simulink subsystem "Drag_Compensator_mk1"  (R2023a)
settings: Solver=VariableStepAuto  StartTime=0.0  StopTime=10.0  RelTol=1e-3
libraries: ros2lib x2

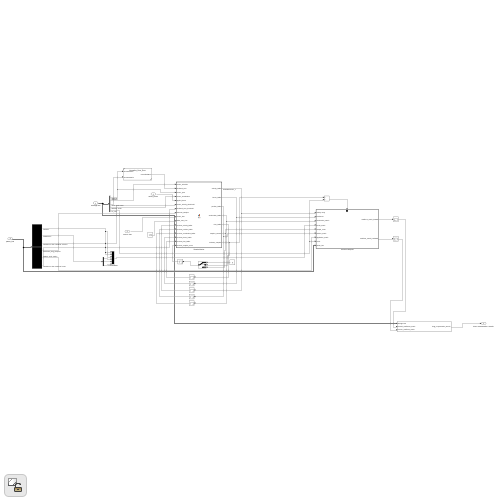
[thumbnail: Simulink's stored preview of the top-level diagram]
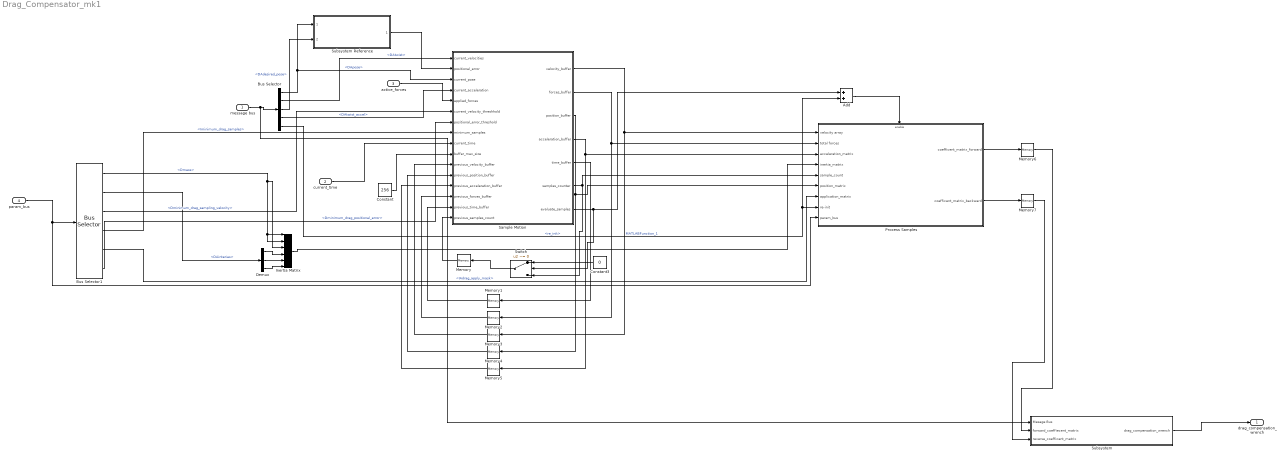
== system Drag_Compensator_mk1 ==
  message bus : Inport
  current_time : Inport  Port=2
  active_forces : Inport  Port=3
  param_bus : Inport  Port=4
  Add : Sum
  Bus Selector : BusSelector  OutputSignals=current_state.DApose,current_state.DAtwist,desired_pose.DAdesired_pose,current_state.DAtwist_accel,re_init
  Bus Selector1 : BusSelector  OutputSignals=Dmass,DAinterias,Dminimum_drag_sampling_velocity,Iminimum_drag_samples,IAdrag_apply_mask,Dminimum_drag_positional_error
  Constant : Constant  Value=256
  Constant3 : Constant  Value=0
  Demux : Demux  Outputs=3
  Inertia Matrix : Mux  Inputs=6
  Memory : Memory
  Memory1 : Memory  InitialCondition=zeros(256,1)
  Memory2 : Memory  InitialCondition=zeros(6,256)
  Memory3 : Memory  InitialCondition=zeros(6,256)
  Memory4 : Memory  InitialCondition=zeros(7,256)
  Memory5 : Memory  InitialCondition=zeros(6,256)
  Memory6 : Memory  InitialCondition=zeros(6,6)
  Memory7 : Memory  InitialCondition=zeros(6,6)
  Process Samples : Subsystem
  Sample Motion : MATLAB Function  TreatAsAtomicUnit=on
  Subsystem : Subsystem
  Subsystem Reference : Subsystem  ReferencedSubsystem=Normalize_Pose_Error
  Switch : Switch  Criteria=u2 ~= 0  SaturateOnIntegerOverflow=off  InputSameDT=off
  drag_compensation_wrench : Outport
  wires:
  Sample Motion/1(velocity_buffer) -> Process Samples/1(velocity array), Memory3/1  "MATLABFunction_1"
  Sample Motion/5(time_buffer) -> Memory1/1
  Sample Motion/6(samples_counter) -> Process Samples/5(sample_count), Switch/3
  Sample Motion/2(forces_buffer) -> Process Samples/2(total forces), Memory2/1
  message bus/1 -> Bus Selector/1, Subsystem/1(Mesage Bus)
  current_time/1 -> Sample Motion/9(current_time)
  Constant/1 -> Sample Motion/10(buffer_max_size)
  Bus Selector/2 -> Sample Motion/1(current_velocities)  "<DAtwist>"
  active_forces/1 -> Sample Motion/5(applied_forces)
  Bus Selector/1 -> Sample Motion/3(current_pose), Subsystem Reference/1  "<DApose>"
  Bus Selector/3 -> Subsystem Reference/2  "<DAdesired_pose>"
  Subsystem Reference/1 -> Sample Motion/2(positional_error)
  Constant3/1 -> Switch/1
  Sample Motion/7(evaluate_samples) -> Add/1, Switch/2
  Switch/1 -> Memory/1
  Memory/1 -> Sample Motion/16(previous_samples_count)
  Memory1/1 -> Sample Motion/15(previous_time_buffer)
  Memory2/1 -> Sample Motion/14(previous_forces_buffer)
  Memory3/1 -> Sample Motion/11(previous_velocity_buffer)
  Sample Motion/3(position_buffer) -> Process Samples/6(position_matrix), Memory4/1
  Memory4/1 -> Sample Motion/12(previous_position_buffer)
  Sample Motion/4(acceleration_buffer) -> Process Samples/3(acceleration_matrix), Memory5/1
  Memory5/1 -> Sample Motion/13(previous_acceleration_buffer)
  Bus Selector/4 -> Sample Motion/4(current_acceleration)  "<DAtwist_accel>"
  param_bus/1 -> Bus Selector1/1, Process Samples/9(param_bus)
  Bus Selector1/2 -> Demux/1  "<DAinterias>"
  Demux/3 -> Inertia Matrix/6
  Demux/2 -> Inertia Matrix/5
  Demux/1 -> Inertia Matrix/4
  Bus Selector1/1 -> Inertia Matrix/3, Inertia Matrix/1, Inertia Matrix/2  "<Dmass>"
  Inertia Matrix/1 -> Process Samples/4(inertia_matrix)
  Process Samples/1(coefficent_matrix_forward) -> Memory6/1
  Bus Selector1/3 -> Sample Motion/6(current_velocity_threshhold)  "<Dminimum_drag_sampling_velocity>"
  Bus Selector1/6 -> Sample Motion/7(positional_error_threshold)  "<Dminimum_drag_positional_error>"
  Bus Selector1/5 -> Process Samples/7(application_matrix)  "<IAdrag_apply_mask>"
  Bus Selector1/4 -> Sample Motion/8(minimum_samples)  "<Iminimum_drag_samples>"
  Bus Selector/5 -> Process Samples/8(re-init), Add/2  "<re_init>"
  Add/1 -> Process Samples/Enable
  Process Samples/2(coefficent_matrix_backward) -> Memory7/1
  Memory6/1 -> Subsystem/2(forward_coeffiecent_matrix)
  Memory7/1 -> Subsystem/3(reverse_coefficent_matrix)
  Subsystem/1(drag_compensation_wrench) -> drag_compensation_wrench/1

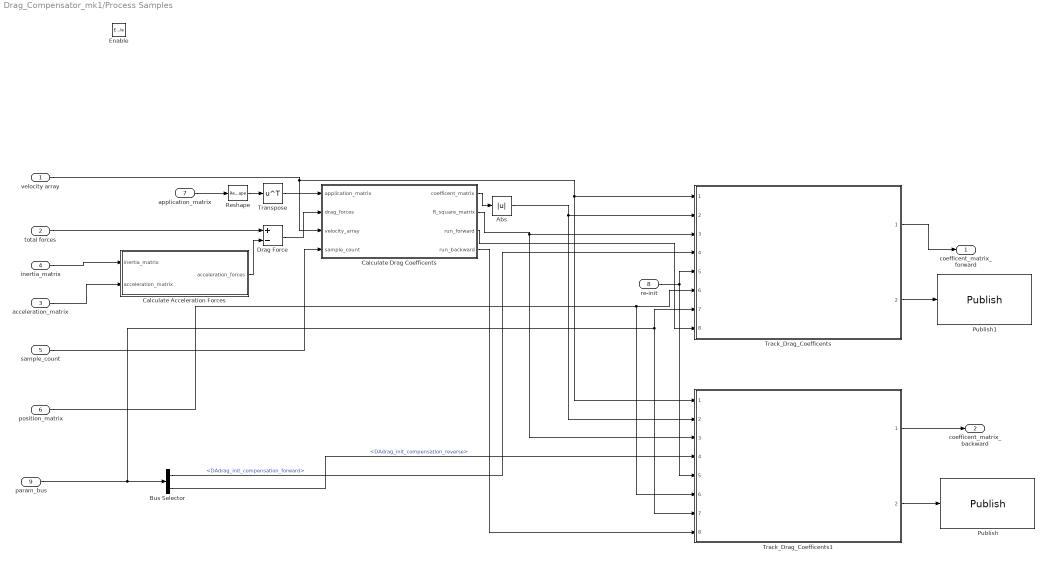
== system Drag_Compensator_mk1/Process Samples ==
  velocity array : Inport
  total forces : Inport  Port=2
  acceleration_matrix : Inport  Port=3
  inertia_matrix : Inport  Port=4
  sample_count : Inport  Port=5
  position_matrix : Inport  Port=6
  application_matrix : Inport  Port=7
  re-init : Inport  Port=8
  param_bus : Inport  Port=9
  Enable : EnablePort
  Abs : Abs  SaturateOnIntegerOverflow=off
  Bus Selector : BusSelector  OutputSignals=DAdrag_init_compensation_forward,DAdrag_init_compensation_reverse
  Calculate Acceleration Forces : MATLAB Function  TreatAsAtomicUnit=on
  Calculate Drag Coefficents : MATLAB Function  TreatAsAtomicUnit=on
  Drag Force : Sum  Inputs=+-
  Publish : ros2lib/Publish  topicSource=Specify your own  topic=/talos/controller/drag_comp/reverse  messageType=geometry_msgs/TwistWithCovariance  QOSHistory=Keep last  QOSDepth=1  QOSReliability=Reliable  QOSDurability=Volatile
  Publish1 : ros2lib/Publish  topicSource=Specify your own  topic=/talos/controller/drag_comp/forward  messageType=geometry_msgs/TwistWithCovariance  QOSHistory=Keep last  QOSDepth=1  QOSReliability=Reliable  QOSDurability=Volatile
  Reshape : Reshape  OutputDimensionality=Customize  OutputDimensions=[6,6]
  Track_Drag_Coefficents : Subsystem  ReferencedSubsystem=Track_Drag_Coefficents
  Track_Drag_Coefficents1 : Subsystem  ReferencedSubsystem=Track_Drag_Coefficents
  Transpose : Math  Operator=transpose
  coefficent_matrix_forward : Outport
  coefficent_matrix_backward : Outport  Port=2
  wires:
  Track_Drag_Coefficents/2 -> Publish1/1
  Track_Drag_Coefficents1/2 -> Publish/1
  Track_Drag_Coefficents1/1 -> coefficent_matrix_backward/1
  Calculate Drag Coefficents/4(run_backward) -> Track_Drag_Coefficents1/8
  Calculate Drag Coefficents/3(run_forward) -> Track_Drag_Coefficents/8
  Bus Selector/2 -> Track_Drag_Coefficents1/4  "<DAdrag_init_compensation_reverse>"
  Bus Selector/1 -> Track_Drag_Coefficents/4  "<DAdrag_init_compensation_forward>"
  param_bus/1 -> Track_Drag_Coefficents/7, Track_Drag_Coefficents1/7, Bus Selector/1
  Track_Drag_Coefficents/1 -> coefficent_matrix_forward/1
  position_matrix/1 -> Track_Drag_Coefficents/6, Track_Drag_Coefficents1/6
  re-init/1 -> Track_Drag_Coefficents/5, Track_Drag_Coefficents1/5
  Calculate Drag Coefficents/2(R_square_matrix) -> Track_Drag_Coefficents/3, Track_Drag_Coefficents1/3
  Abs/1 -> Track_Drag_Coefficents/2, Track_Drag_Coefficents1/2
  Transpose/1 -> Calculate Drag Coefficents/1(application_matrix)
  Reshape/1 -> Transpose/1
  velocity array/1 -> Track_Drag_Coefficents/1, Track_Drag_Coefficents1/1, Calculate Drag Coefficents/3(velocity_array)
  Calculate Drag Coefficents/1(coefficent_matrix) -> Abs/1
  sample_count/1 -> Calculate Drag Coefficents/4(sample_count)
  inertia_matrix/1 -> Calculate Acceleration Forces/1(inertia_matrix)
  total forces/1 -> Drag Force/1
  acceleration_matrix/1 -> Calculate Acceleration Forces/2(acceleration_matrix)
  Drag Force/1 -> Calculate Drag Coefficents/2(drag_forces)
  Calculate Acceleration Forces/1(acceleration_forces) -> Drag Force/2
  application_matrix/1 -> Reshape/1

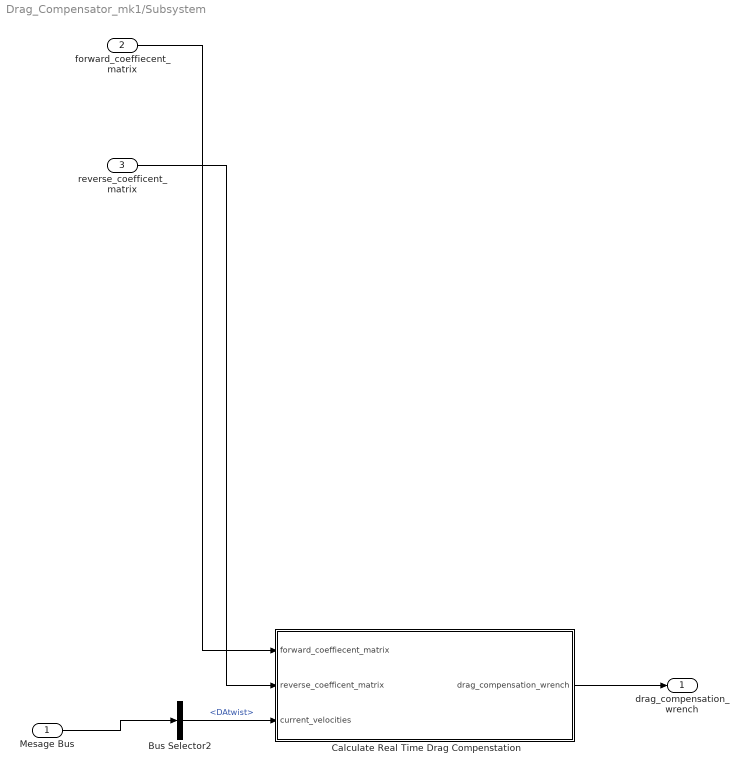
== system Drag_Compensator_mk1/Subsystem ==
  Mesage Bus : Inport
  forward_coeffiecent_matrix : Inport  Port=2
  reverse_coefficent_matrix : Inport  Port=3
  Bus Selector2 : BusSelector  OutputSignals=current_state.DAtwist
  Calculate Real Time Drag Compenstation : MATLAB Function  TreatAsAtomicUnit=on
  drag_compensation_wrench : Outport
  wires:
  forward_coeffiecent_matrix/1 -> Calculate Real Time Drag Compenstation/1(forward_coeffiecent_matrix)
  Calculate Real Time Drag Compenstation/1(drag_compensation_wrench) -> drag_compensation_wrench/1
  reverse_coefficent_matrix/1 -> Calculate Real Time Drag Compenstation/2(reverse_coefficent_matrix)
  Mesage Bus/1 -> Bus Selector2/1
  Bus Selector2/1 -> Calculate Real Time Drag Compenstation/3(current_velocities)  "<DAtwist>"

== matlab function Drag_Compensator_mk1/Sample Motion ==
function [velocity_buffer, forces_buffer, position_buffer, acceleration_buffer, time_buffer, samples_counter, evaluate_samples] = fcn(current_velocities, positional_error, current_pose, current_acceleration, applied_forces, current_velocity_threshhold, positional_error_threshold, minimum_samples, current_time, buffer_max_size, previous_velocity_buffer, previous_position_buffer,  previous_acceleration_buffer, previous_forces_buffer, previous_time_buffer, previous_samples_count)

%determine if now is a good time for sampling
linear_velocity = norm(current_velocities(1:3));
linear_positional_error = norm(positional_error(1:3));

%initialize the variables
velocity_buffer = previous_velocity_buffer(1:6, 1:256);
position_buffer = previous_position_buffer(1:7, 1:256);
forces_buffer = previous_forces_buffer(1:6, 1:256);
acceleration_buffer = previous_acceleration_buffer(1:6, 1:256);
time_buffer = previous_time_buffer(1:256);

if(linear_velocity > current_velocity_threshhold && linear_positional_error > positional_error_threshold)
    %record samples

    samples_counter = previous_samples_count + 1;

    %add samples to the front of the buffers
    velocity_buffer(1:6, samples_counter) = current_velocities;
    position_buffer(1:7, samples_counter) = current_pose;
    forces_buffer(1:6, samples_counter) = applied_forces;
    time_buffer(samples_counter) = current_time;  
    acceleration_buffer(1:6, samples_counter) = current_acceleration;

    if(samples_counter == buffer_max_size)
        evaluate_samples = true;
    else
        evaluate_samples = false;
    end

    return

elseif(previous_samples_count > minimum_samples)
    %done recording - eval now

    evaluate_samples = true;
    samples_counter = previous_samples_count;

    return
end

velocity_buffer = velocity_buffer .* 0;
position_buffer = position_buffer .* 0;
forces_buffer = forces_buffer .* 0;
time_buffer = time_buffer .* 0;
acceleration_buffer = acceleration_buffer .* 0;

samples_counter = 0;
evaluate_samples = false;

== matlab function Drag_Compensator_mk1/Process Samples/Calculate Drag Coefficents ==
function [coefficent_matrix, R_square_matrix, run_forward, run_backward] = fcn(application_matrix, drag_forces, velocity_array, sample_count)

coefficent_matrix = zeros(6,6);
R_square_matrix = zeros(6,6);

    for correction_axis = 1:6
        for motion_axis = 1:6
            if(application_matrix(correction_axis, motion_axis))
                [coefficent_matrix(correction_axis, motion_axis), R_square_matrix(correction_axis, motion_axis)] = fit_cruve(velocity_array(motion_axis, 1:sample_count), drag_forces(correction_axis, 1:sample_count));
            end
        end
    end

run_forward = sign(mean(velocity_array, 2)) > 0;
run_backward = ~run_forward;
end


function [coeffiecent, R_squared] = fit_cruve(vel_data, drag_data)

    x_matrix = vel_data' .^ 2;
    y_vector = drag_data';

    coeffiecent = inv(x_matrix' * x_matrix) * x_matrix' * y_vector;

    original_sum_of_sqaures = sum(drag_data .^ 2);
    adjusted_sum_of_sqaures = sum((drag_data - coeffiecent * vel_data .^ 2) .^ 2);

    R_squared = 1 - adjusted_sum_of_sqaures / original_sum_of_sqaures;
end

== matlab function Drag_Compensator_mk1/Process Samples/Calculate Acceleration Forces ==
function acceleration_forces = fcn(inertia_matrix, acceleration_matrix)

acceleration_forces = zeros(6, 256);

for i=1:6
   acceleration_forces(i,:) = inertia_matrix(i) * acceleration_matrix(i,:); 
end

== matlab function Drag_Compensator_mk1/Subsystem/Calculate Real Time Drag Compenstation ==
function drag_compensation_wrench = fcn(forward_coeffiecent_matrix, reverse_coefficent_matrix, current_velocities)

combined_coefficent_matrix = zeros(6,6);

for motion_axis = 1:6

    if(current_velocities(motion_axis) > 0)
        combined_coefficent_matrix(:, motion_axis) = forward_coeffiecent_matrix(:, motion_axis);
    else
        combined_coefficent_matrix(:, motion_axis) = reverse_coefficent_matrix(:, motion_axis);
    end
end

drag_compensation_wrench = combined_coefficent_matrix * (abs(current_velocities) .* current_velocities);
